simulink model "buck_digital"  (R2020a)
settings: Solver=VariableStepAuto  StartTime=0.0  StopTime=0.05  RelTol=1e-3
libraries: powerlib x13, simulink_extras x1, discretizing x1, powerlib_meascontrol x1
settings Model: Creator=ayanc  LastModifiedBy=ayanc
settings SolverCC: ZeroCrossAlgorithm=Adaptive
settings DebuggingCC: IgnoredZcDiagnostic=none

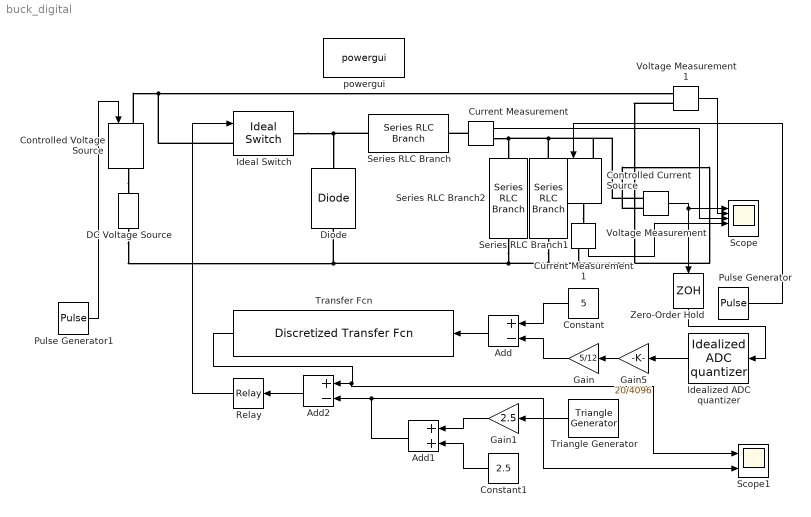
== system buck_digital ==
  Add : Sum  Inputs=+-
  Add1 : Sum
  Add2 : Sum  Inputs=+-
  Constant : Constant  Value=5
  Constant1 : Constant  Value=2.5
  Controlled Current Source : powerlib/Electrical Sources/Controlled Current Source  Initialize=on  Source_Type=DC  Amplitude=5  Phase=0  Frequency=0  Measurements=None
  Controlled Voltage Source : powerlib/Electrical Sources/Controlled Voltage Source  Initialize=on  Source_Type=AC  Amplitude=0  Phase=0  Frequency=0  Measurements=None
  Current Measurement : powerlib/Measurements/Current Measurement  PhasorSimulation=off  OutputType=Complex  PSBequivalent=0
  Current Measurement1 : powerlib/Measurements/Current Measurement  PhasorSimulation=off  OutputType=Complex  PSBequivalent=0
  DC Voltage Source : powerlib/Electrical Sources/DC Voltage Source  Amplitude=22  Measurements=None
  Diode : powerlib/Power Electronics/Diode  Ron=0  Lon=0  Vf=0  IC=0  UseSnubber=0  Rs=inf  Cs=0  Measurements=off
  Gain : Gain  Gain=5/12
  Gain1 : Gain  Gain=2.5
  Gain5 : Gain  Gain=20/4096
  Ideal Switch : powerlib/Power Electronics/Ideal Switch  Ron=0  Lon=0  IC=0  Rs=inf  Cs=inf  Measurements=off
  Idealized ADC quantizer : simulink_extras/Additional Discrete/Idealized ADC quantizer  NumberOfConverterBits=12  Vmin=0  Vmax=20  OutputDataType=int16  OutputNegativeValues=off
  Pulse Generator : DiscretePulseGenerator  PulseType=Time based  Amplitude=5  Period=0.02  PulseWidth=50  PhaseDelay=0.01
  Pulse Generator1 : DiscretePulseGenerator  PulseType=Time based  Amplitude=5  Period=0.02  PulseWidth=50  PhaseDelay=0.005
  Relay : Relay
  Scope : Scope  NumInputPorts=5
  Scope1 : Scope  NumInputPorts=2
  Series RLC Branch : powerlib/Elements/Series RLC Branch  LConnTagsString=__new0  RConnTagsString=__new0  BranchType=L  Resistance=1  Inductance=5e-06  SetiL0=off  InitialCurrent=0  Capacitance=1e-6  Setx0=off  InitialVoltage=0  Measurements=None
  Series RLC Branch1 : powerlib/Elements/Series RLC Branch  LConnTagsString=__new0  RConnTagsString=__new0  BranchType=R  Resistance=1.2  Inductance=1e-3  SetiL0=off  InitialCurrent=0  Capacitance=1e-6  Setx0=off  InitialVoltage=0  Measurements=None
  Series RLC Branch2 : powerlib/Elements/Series RLC Branch  LConnTagsString=__new0  RConnTagsString=__new0  BranchType=C  Resistance=1  Inductance=1e-3  SetiL0=off  InitialCurrent=0  Capacitance=40e-6  Setx0=off  InitialVoltage=0  Measurements=None
  Transfer Fcn : discretizing/Discretized Transfer Fcn  Numerator=100*[4.61696 1767103.018 9.947609866e10]  Denominator=[0.0019 68582.41276 0]  AbsTol=auto  SampleTime=1e-7  method=zoh  Wc=1
      settings: SourceProductBaseCode=SL
  Triangle Generator : powerlib_meascontrol/Pulse & Signal Generators/Triangle Generator  Freq=500e3  Phase=90  Ts=0
  Voltage Measurement : powerlib/Measurements/Voltage Measurement  PhasorSimulation=off  OutputType=Complex  PSBequivalent=0
  Voltage Measurement1 : powerlib/Measurements/Voltage Measurement  PhasorSimulation=off  OutputType=Complex  PSBequivalent=0
  Zero-Order Hold : ZeroOrderHold  SampleTime=1e-7
  powergui : powerlib/powergui  Priority=1  SimulationMode=Continuous  SampleTime=50e-6  frequency=60  Iterations=50  frequencyindice=0  Pbase=100e6  ErrMax=1e-4  UnitsV=kV  UnitsW=MW  buscounter=0  FunctionMessages=off  echomessages=off  EnableUseOfTLC=off  CurrentSourceSwitches=off  DisableSnubberDevices=off  DisableRonSwitches=off  DisableVfSwitches=off  DisplayEquations=off  AutomaticDiscreteSolvers=off  SolverType=Tustin/Backward Euler (TBE)  Interpol=off  ExternalGateDelay=off  methode=off  Ts=100  x0status=blocks  SPID=on  SwTol=0  HookPort=off  NonlinearTolerance=1e-4  nMaxIteration=100  ContinueOnMaxIteration=off  RestoreLinks=warning  ResistiveCurrentMeasurement=off  Frange=[0:2:500]  Ylog=off  Xlog=on  ShowGrid=off  save=off  variable=ZData  structure=0  ZoomFFT=off  StartTime=0.0  cycles=1  DisplayStyle=1  fundamental=60  FreqAxis=off  MaxFrequency=1000  frequencyindicesteady=1  RmsSteady=1  display=off
  wires:
  Voltage Measurement/1 -> Zero-Order Hold/1, Scope/1
  Gain/1 -> Add/2
  Constant/1 -> Add/1
  Add/1 -> Transfer Fcn/1
  Triangle Generator/1 -> Gain1/1
  Gain1/1 -> Add1/1
  Constant1/1 -> Add1/2
  Transfer Fcn/1 -> Scope1/1, Add2/1
  Add1/1 -> Add2/2, Scope1/2
  Add2/1 -> Relay/1
  Voltage Measurement1/1 -> Scope/2
  Current Measurement/1 -> Scope/3
  Current Measurement1/1 -> Scope/4
  Pulse Generator/1 -> Controlled Current Source/1
  Relay/1 -> Ideal Switch/1
  Pulse Generator1/1 -> Controlled Voltage Source/1
  Gain5/1 -> Gain/1
  Idealized ADC quantizer/1 -> Gain5/1
  Zero-Order Hold/1 -> Idealized ADC quantizer/1
  connections:
  Series RLC Branch/LConn1 -- Diode/RConn1 -- Ideal Switch/RConn1
  DC Voltage Source/LConn1 -- Voltage Measurement1/LConn2 -- Voltage Measurement/LConn2 -- Current Measurement1/RConn1 -- Series RLC Branch1/RConn1 -- Series RLC Branch2/RConn1 -- Diode/LConn1
  Controlled Current Source/LConn1 -- Voltage Measurement/LConn1 -- Series RLC Branch1/LConn1 -- Series RLC Branch2/LConn1 -- Current Measurement/RConn1
  Current Measurement/LConn1 -- Series RLC Branch/RConn1
  Ideal Switch/LConn1 -- Controlled Voltage Source/LConn1 -- Voltage Measurement1/LConn1
  Controlled Current Source/RConn1 -- Current Measurement1/LConn1
  Controlled Voltage Source/RConn1 -- DC Voltage Source/RConn1
